simulink model "Ex2_MotorResponse"  (R2025b)
settings: Solver=FixedStepAuto  StartTime=0.0  StopTime=15  RelTol=1e-3  EnableMultiTasking=on
undefined symbols (not defined in the file): motor_param
libraries: simulink x4, arduinolib x4, SigiLib x1
settings Model: ExtModeTrigDuration=2  Creator=resjoehr  LastModifiedBy=resjoehr
settings OptimizationCC: EnhancedBackFolding=on  PassReuseOutputArgsAs=Individual arguments  ZeroExternalMemoryAtStartup=off  ZeroInternalMemoryAtStartup=off  MaxStackSize=64  OptimizeBlockOrder=speed  DifferentSizesBufferReuse=on  OptimizationCustomize=off  EfficientTunableParamExpr=on
settings DebuggingCC: ParameterTunabilityLossMsg=error
settings HardwareCC: ProdBitPerInt=16.0  ProdBitPerPointer=16.0  ProdBitPerSizeT=16.0  ProdBitPerPtrDiffT=16.0  ProdLargestAtomicFloat=None  ProdWordSize=8.0  ProdHWDeviceType=Atmel->AVR
settings SFSimCC: MATLABDynamicMemAlloc=off
settings RTWCC: SystemTargetFile=ert.tlc  HardwareBoard=Arduino Leonardo  TemplateMakefile=ert_default_tmf  Toolchain=Arduino AVR  BuildConfiguration=Faster Runs  GPUComputeCapability=3.5  Description=Embedded Coder
settings CodeAppCC: ForceParamTrailComments=on  IgnoreCustomStorageClasses=off  OperatorAnnotations=on  SimulinkDataObjDesc=on  SFDataObjDesc=on  InsertBlockDesc=on
settings ERTTargetCC: ExtModeTransport=3.0  ExtModeStaticAlloc=on  ExtModeAutomaticAllocSize=off  ExtModeStaticAllocSize=250.0  ExtModeMexFile=ext_xcp  ExtModeIntrfLevel=Level2 - Open  InlinedParameterPlacement=Hierarchical  DynamicArrayContainerType=coder::array  SupportContinuousTime=on  SupportVariableSizeSignals=on

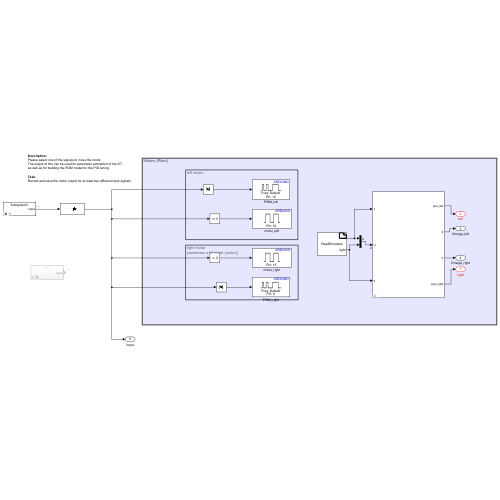
[thumbnail: Simulink's stored preview of the top-level diagram]
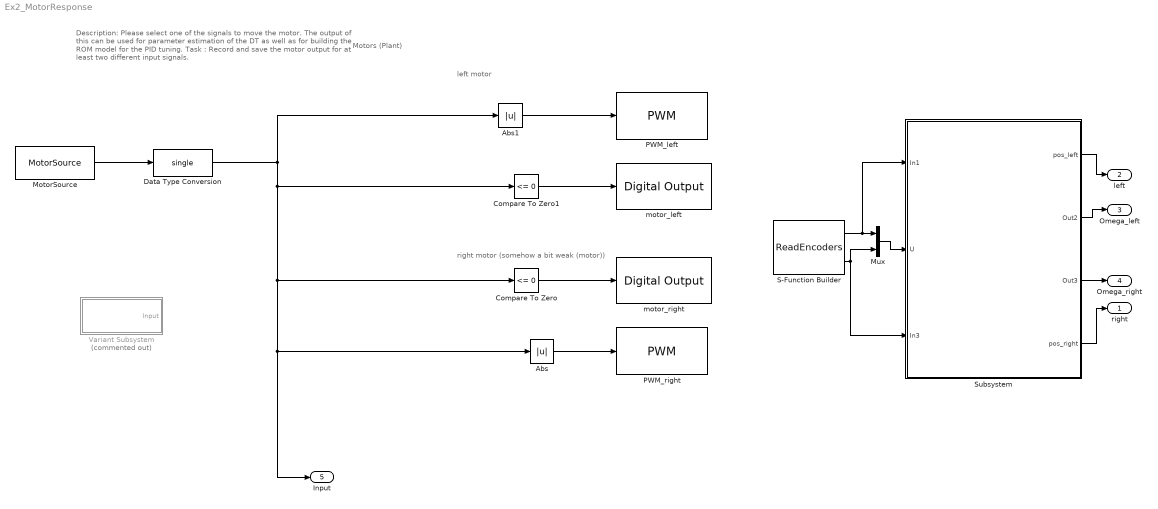
== system Ex2_MotorResponse ==
  note: Description:
      | Please select one of the signals to move the motor.
      | The output of this can be used for parameter estimation of the DT
      | as well as for building the ROM model for the PID tuning.
      |
      | Task :
      | Record and save the motor output for at least two different input signals.
  note: Motors (Plant)
  note: left motor
  note: right motor
      | (somehow a bit weak (motor))
  Abs : Abs  SaturateOnIntegerOverflow=off
  Abs1 : Abs  OutDataTypeStr=single  SaturateOnIntegerOverflow=off
  Compare To Zero : simulink/Logic and Bit Operations/Compare To Zero  relop=<=  OutDataTypeStr=boolean
  Compare To Zero1 : simulink/Logic and Bit Operations/Compare To Zero  relop=<=  OutDataTypeStr=boolean
  Data Type Conversion : DataTypeConversion  OutDataTypeStr=single  SaturateOnIntegerOverflow=off  RndMeth=Floor
  MotorSource : SigiLib/MotorSource  LabelModeActiveChoice=Square  amp=120
  Mux : Mux  Inputs=2
  PWM_left : arduinolib/PWM  pinNumber=10  frequencyType=Default  desiredFrequency=1410  achievableFrequency=1409.9401
  PWM_right : arduinolib/PWM  pinNumber=9  frequencyType=Default  desiredFrequency=1410  achievableFrequency=1409.9401
  S-Function Builder : S-Function  InitFcn=try, set_param(gcb,'FunctionName','ReadEncoders'), end  FunctionName=ReadEncoders  SFunctionModules=ReadEncoders_wrapper.cpp  SFunctionDeploymentMode=off  EnableBusSupport=off  mask(S-Function Builder){}
      mask help: Simulink:masks:SFunctionBuilder_MD
      mask init:
      | val = [[.9  0.75 0.75 1 1 .9 .9 1]',[1 1 0.75 0.75 .9 .9 1 .9]'];try , sys = get_param(gcb,'SfunBuilderFcnName');if isempty(sys), sys = get_param(gcb,'FunctionName'); end,catch, sys = get_param(gcb,'FunctionName'); end
      settings: CopyFcn=set_param(gcbh,'LinkStatus','none')  PreSaveFcn=try, set_param(gcb,'FunctionName','ReadEncoders'), end  OpenFcn=sfunctionwizard(gcbh)
      mask Display:
      | plot(val(:,1),val(:,2))
      | disp(sys)
      | port_label('output',1,'left')
      | port_label('output',2,'right')
  Subsystem : Subsystem  mask{gear_box=motor_param.gear_ratio, motor_gear=motor_param.motor_ratio}
      mask prompts: gear_box "Gear box ratio:"; motor_gear "Motor gear ratio:"
  Variant Subsystem : Subsystem  Commented=on  Variant=on  VariantControlMode=label  LabelModeActiveChoice=Square
  motor_left : arduinolib/Digital Output  pinNumber=16  Direction=output  blockPlatform=arduino
  motor_right : arduinolib/Digital Output  pinNumber=15  Direction=output  blockPlatform=arduino
  right : Outport  OutDataTypeStr=single
  left : Outport  Port=2  OutDataTypeStr=single
  Omega_left : Outport  Port=3
  Omega_right : Outport  Port=4
  Input : Outport  Port=5
  wires:
  Compare To Zero1/1 -> motor_left/1
  Abs/1 -> PWM_right/1
  Compare To Zero/1 -> motor_right/1
  Abs1/1 -> PWM_left/1
  S-Function Builder/1 -> Subsystem/1(In1), Mux/1
  S-Function Builder/2 -> Subsystem/3(In3), Mux/2
  MotorSource/1 -> Data Type Conversion/1
  Mux/1 -> Subsystem/2(U)
  Subsystem/1(pos_left) -> left/1
  Subsystem/2(Out2) -> Omega_left/1
  Subsystem/3(Out3) -> Omega_right/1
  Subsystem/4(pos_right) -> right/1
  Data Type Conversion/1 -> Abs/1, Input/1, Compare To Zero/1, Compare To Zero1/1, Abs1/1

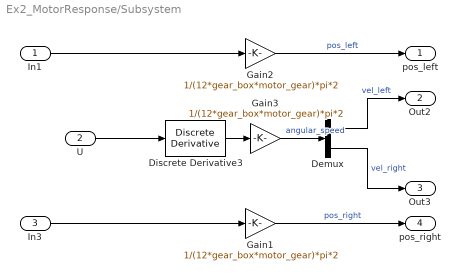
== system Ex2_MotorResponse/Subsystem ==
  In1 : Inport
  U : Inport  Port=2
  In3 : Inport  Port=3
  Demux : Demux  Outputs=2
  Discrete Derivative3 : simulink/Discrete/Discrete Derivative  gainval=1  ICPrevScaledInput=0.0  OutMin=[]  OutMax=[]  OutDataType=fixdt(1, 16)  OutScaling=2^-10  DoSatur=off
  Gain1 : Gain  Gain=1/(12*gear_box*motor_gear)*pi*2  OutDataTypeStr=single
  Gain2 : Gain  Gain=1/(12*gear_box*motor_gear)*pi*2
  Gain3 : Gain  Gain=1/(12*gear_box*motor_gear)*pi*2
  pos_left : Outport
  Out2 : Outport  Port=2
  Out3 : Outport  Port=3
  pos_right : Outport  Port=4
  wires:
  In3/1 -> Gain1/1
  Discrete Derivative3/1 -> Gain3/1
  U/1 -> Discrete Derivative3/1
  Demux/1 -> Out2/1  "vel_left"
  Gain3/1 -> Demux/1  "angular_speed"
  Demux/2 -> Out3/1  "vel_right"
  Gain2/1 -> pos_left/1  "pos_left"
  In1/1 -> Gain2/1
  Gain1/1 -> pos_right/1  "pos_right"

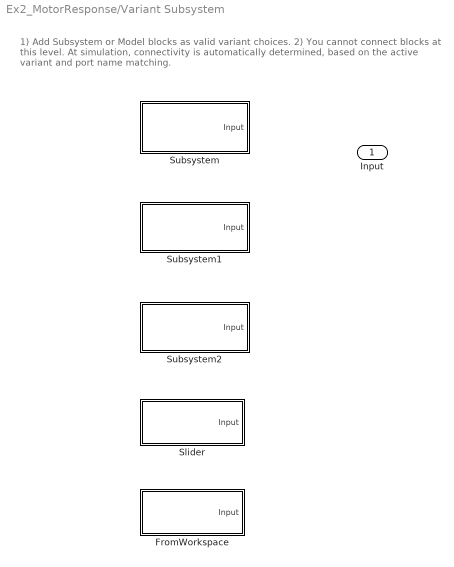
== system Ex2_MotorResponse/Variant Subsystem ==
  note: 1) Add Subsystem or Model blocks as valid variant choices.
      | 2) You cannot connect blocks at this level. At simulation, connectivity is automatically
      | determined, based on the active variant and port name matching.
  FromWorkspace : Subsystem  VariantControl=FromWorkspace
  Slider : Subsystem  VariantControl=Slider
  Subsystem : Subsystem  VariantControl=Custom
  Subsystem1 : Subsystem  VariantControl=Square
  Subsystem2 : Subsystem  VariantControl=Ramp
  Input : Outport

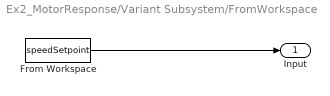
== system Ex2_MotorResponse/Variant Subsystem/FromWorkspace ==
  From Workspace : FromWorkspace  VariableName=speedSetpoint
  Input : Outport
  wires:
  From Workspace/1 -> Input/1

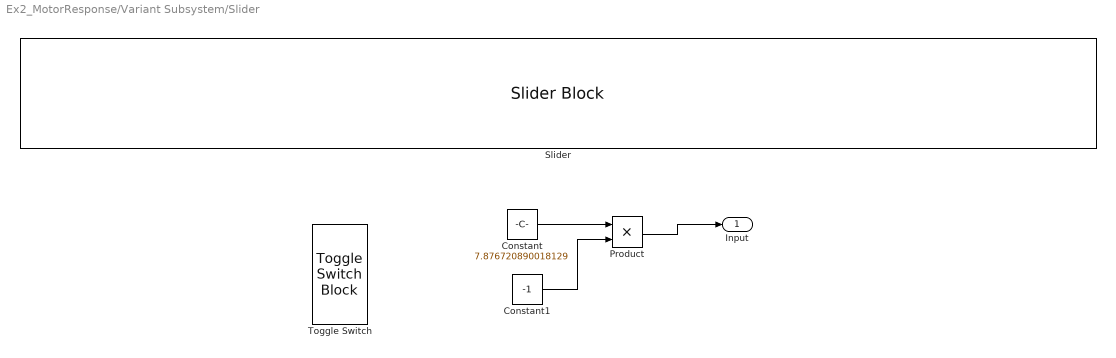
== system Ex2_MotorResponse/Variant Subsystem/Slider ==
  Constant : Constant  Value=7.876720890018129
  Constant1 : Constant  Value=-1
  Product : Product
  Slider : SliderBlock  TickInterval=5
  Toggle Switch : ToggleSwitchBlock
  Input : Outport
  wires:
  Constant/1 -> Product/1
  Product/1 -> Input/1
  Constant1/1 -> Product/2

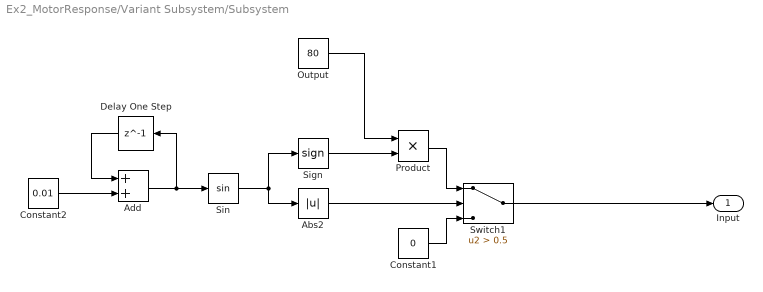
== system Ex2_MotorResponse/Variant Subsystem/Subsystem ==
  Abs2 : Abs  OutDataTypeStr=single  SaturateOnIntegerOverflow=off
  Add : Sum  OutDataTypeStr=single
  Constant1 : Constant  Value=0  OutDataTypeStr=single  SampleTime=0.01
  Constant2 : Constant  Value=0.01
  Delay One Step : Delay  DelayLength=1  SampleTime=0.01
  Output : Constant  Value=80  OutDataTypeStr=single  SampleTime=0.01
  Product : Product
  Sign : Signum
  Sin : Trigonometry  OutputSignalType=real
  Switch1 : Switch  Criteria=u2 > Threshold  Threshold=0.5  SaturateOnIntegerOverflow=off  InputSameDT=off
  Input : Outport
  wires:
  Switch1/1 -> Input/1
  Abs2/1 -> Switch1/2
  Add/1 -> Delay One Step/1, Sin/1
  Sin/1 -> Abs2/1, Sign/1
  Output/1 -> Product/1
  Product/1 -> Switch1/1
  Sign/1 -> Product/2
  Constant2/1 -> Add/2
  Delay One Step/1 -> Add/1
  Constant1/1 -> Switch1/3

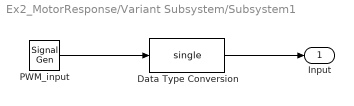
== system Ex2_MotorResponse/Variant Subsystem/Subsystem1 ==
  Data Type Conversion : DataTypeConversion  OutDataTypeStr=single  SaturateOnIntegerOverflow=off  RndMeth=Floor
  PWM_input : SignalGenerator  WaveForm=square  Amplitude=120  Frequency=0.3
  Input : Outport
  wires:
  PWM_input/1 -> Data Type Conversion/1
  Data Type Conversion/1 -> Input/1

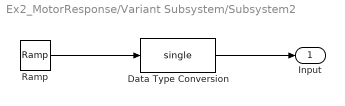
== system Ex2_MotorResponse/Variant Subsystem/Subsystem2 ==
  Data Type Conversion : DataTypeConversion  OutDataTypeStr=single  SaturateOnIntegerOverflow=off  RndMeth=Floor
  Ramp : simulink/Sources/Ramp  slope=25.5  start=0  InitialOutput=0
  Input : Outport
  wires:
  Ramp/1 -> Data Type Conversion/1
  Data Type Conversion/1 -> Input/1
